simulink model "plant"  (R2021b)
settings: Solver=VariableStepAuto  StartTime=0.0  StopTime=10.0  RelTol=1e-3
settings Model: Creator=DAUIN-Win10  LastModifiedBy=sagai

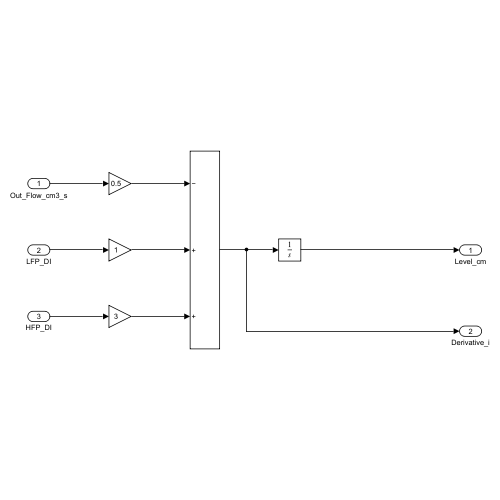
[thumbnail: Simulink's stored preview of the top-level diagram]
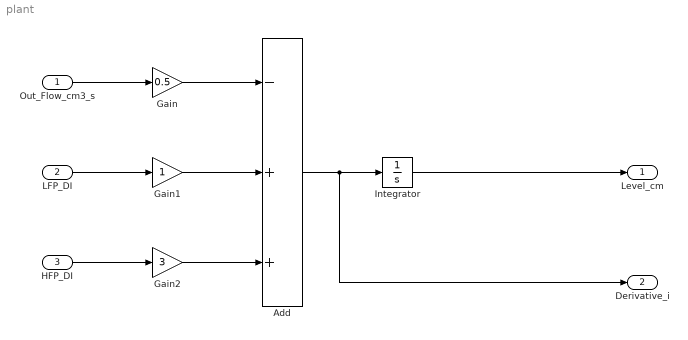
== system plant ==
  Out_Flow_cm3_s : Inport
  LFP_DI : Inport  Port=2  OutDataTypeStr=boolean
  HFP_DI : Inport  Port=3  OutDataTypeStr=boolean
  Add : Sum  Inputs=-++
  Gain : Gain  Gain=0.5
  Gain1 : Gain
  Gain2 : Gain  Gain=3
  Integrator : Integrator  InitialCondition=130
  Level_cm : Outport
  Derivative_i : Outport  Port=2
  wires:
  Out_Flow_cm3_s/1 -> Gain/1
  Integrator/1 -> Level_cm/1
  Gain/1 -> Add/1
  LFP_DI/1 -> Gain1/1
  HFP_DI/1 -> Gain2/1
  Add/1 -> Derivative_i/1, Integrator/1
  Gain1/1 -> Add/2
  Gain2/1 -> Add/3
